simulink model "Exercise74"  (R2023b)
settings: Solver=VariableStepAuto  StartTime=0.0  StopTime=10.0  RelTol=1e-3
libraries: simulink x8
settings Model: Creator=jsonm  LastModifiedBy=jsonm

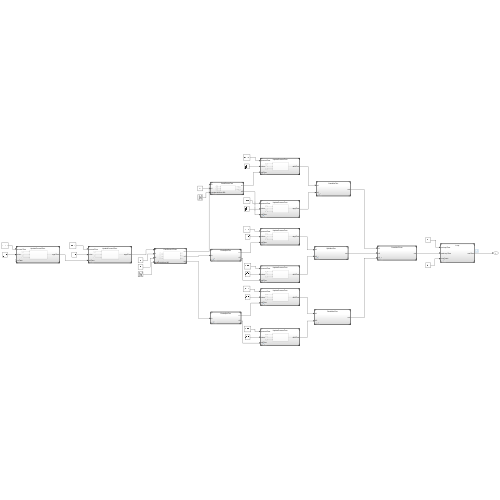
[thumbnail: Simulink's stored preview of the top-level diagram]
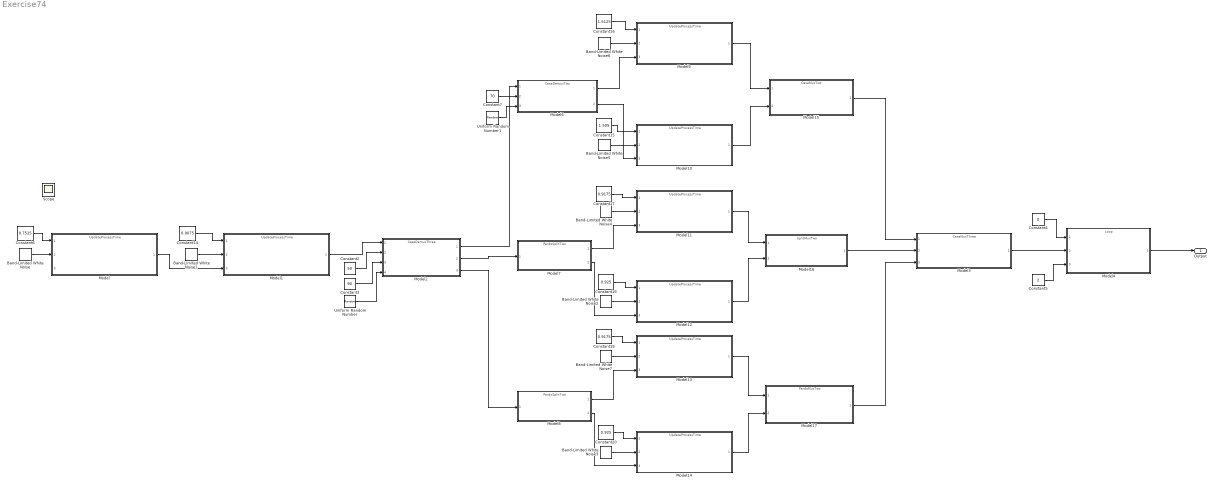
== system Exercise74 ==
  Band-Limited White Noise{,1..7} (8 alike) : simulink/Sources/Band-Limited White Noise  Cov=[0.1]  Ts=0.1  seed=[23341]
  Constant14 : Constant  Value=0.0075
  Constant15 : Constant  Value=1.505
  Constant16 : Constant  Value=1.5125
  Constant17 : Constant  Value=0.9175
  Constant18 : Constant  Value=0.9175
  Constant19 : Constant  Value=0.925
  Constant2 : Constant  Value=50
  Constant20 : Constant  Value=0.925
  Constant3 : Constant  Value=90
  Constant4 : Constant  Value=0
  Constant5 : Constant  Value=2
  Constant6 : Constant  Value=0.7525
  Constant7 : Constant  Value=70
  Model{,1,9..14} (8 alike) : ModelReference  ModelNameDialog=UpdateProcessTime.slx  SimulationMode=Normal  ModelReferenceVersion=1.6
  Model15 : ModelReference  ModelNameDialog=CaseMuxTwo.slx  SimulationMode=Normal  ModelReferenceVersion=1.6
  Model16 : ModelReference  ModelNameDialog=SplitMuxTwo.slx  SimulationMode=Normal  ModelReferenceVersion=1.4
  Model17 : ModelReference  ModelNameDialog=PardoMuxTwo.slx  SimulationMode=Normal  ModelReferenceVersion=1.5
  Model2 : ModelReference  ModelNameDialog=CaseDemuxThree.slx  SimulationMode=Normal  ModelReferenceVersion=1.15
  Model3 : ModelReference  ModelNameDialog=CaseMuxThree.slx  SimulationMode=Normal  ModelReferenceVersion=1.9
  Model4 : ModelReference  ModelNameDialog=Loop.slx  SimulationMode=Normal  ModelReferenceVersion=1.1
  Model6 : ModelReference  ModelNameDialog=CaseDemuxTwo.slx  SimulationMode=Normal  ModelReferenceVersion=1.13
  Model7 : ModelReference  ModelNameDialog=PardoSplitTwo.slx  SimulationMode=Normal  ModelReferenceVersion=1.3
  Model8 : ModelReference  ModelNameDialog=PardoSplitTwo.slx  SimulationMode=Normal  ModelReferenceVersion=1.3
  Uniform Random Number : UniformRandomNumber  Minimum=0  Maximum=100  SampleTime=0.1
  Uniform Random Number1 : UniformRandomNumber  Minimum=0  Maximum=100  Seed=1  SampleTime=0.1
  Output : Outport
  Scope : Scope
  wires:
  Model/1 -> Model1/3
  Model1/1 -> Model2/1
  Constant2/1 -> Model2/2
  Constant3/1 -> Model2/3
  Model2/1 -> Model6/1
  Constant7/1 -> Model6/2
  Model2/2 -> Model7/1
  Model2/3 -> Model8/1
  Model6/1 -> Model9/3
  Model6/2 -> Model10/3
  Model7/1 -> Model11/3
  Model7/2 -> Model12/3
  Model8/1 -> Model13/3
  Model8/2 -> Model14/3
  Model9/1 -> Model15/1
  Model10/1 -> Model15/2
  Model11/1 -> Model16/1
  Model12/1 -> Model16/2
  Model13/1 -> Model17/1
  Model14/1 -> Model17/2
  Model15/1 -> Model3/1
  Model16/1 -> Model3/2
  Model17/1 -> Model3/3
  Model3/1 -> Model4/2
  Model4/1 -> Output/1
  Constant4/1 -> Model4/1
  Constant5/1 -> Model4/3
  Constant6/1 -> Model/1
  Constant14/1 -> Model1/1
  Constant15/1 -> Model10/1
  Constant16/1 -> Model9/1
  Constant17/1 -> Model11/1
  Constant18/1 -> Model13/1
  Constant19/1 -> Model12/1
  Constant20/1 -> Model14/1
  Band-Limited White Noise/1 -> Model/2
  Band-Limited White Noise1/1 -> Model1/2
  Band-Limited White Noise2/1 -> Model12/2
  Band-Limited White Noise3/1 -> Model14/2
  Band-Limited White Noise4/1 -> Model11/2
  Band-Limited White Noise5/1 -> Model10/2
  Band-Limited White Noise6/1 -> Model9/2
  Band-Limited White Noise7/1 -> Model13/2
  Uniform Random Number/1 -> Model2/4
  Uniform Random Number1/1 -> Model6/3
